simulink model "PI_continuo"  (R2012b)
settings: Solver=ode45  StartTime=0.0  StopTime=100  RelTol=1e-3
settings Model: Creator=Walter  LastModifiedBy=Walter

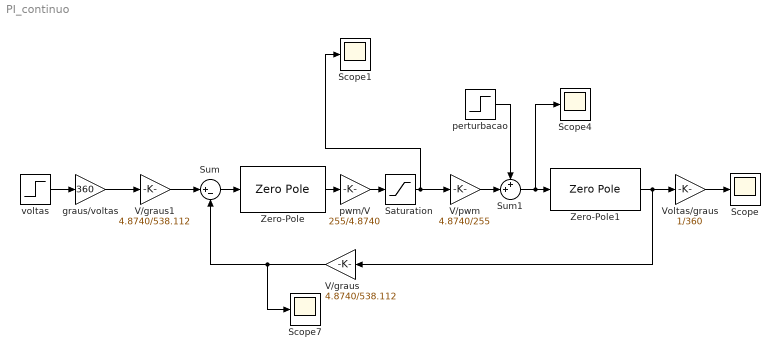
== system PI_continuo ==
  Saturation : Saturate  UpperLimit=255  LowerLimit=-255
  Scope{,1,4,7} (4 alike) : Scope
      Scope settings: TimeRange=60  YMin=2.5  YMax=6.5
      Scope1 settings: TimeRange=100
      Scope4 settings: SaveName=ScopeData4
      Scope7 settings: SaveName=ScopeData7
  Sum : Sum  Inputs=|+-
  Sum1 : Sum  Inputs=++|
  V/graus : Gain  Gain=4.8740/538.112
  V/graus1 : Gain  Gain=4.8740/538.112
  V/pwm : Gain  Gain=4.8740/255
  Voltas/graus : Gain  Gain=1/360
  Zero-Pole : ZeroPole  Zeros=[ -2.54]  Poles=[0]  Gain=[0.94]
  Zero-Pole1 : ZeroPole  Zeros=[]  Poles=[0 -35.7143]  Gain=[3943.0214]
  graus/voltas : Gain  Gain=360
  perturbacao : Step  After=0  SampleTime=0
  pwm/V : Gain  Gain=255/4.8740
  "voltas " : Step  Time=0  After=20  SampleTime=0
  wires:
  Sum/1 -> Zero-Pole/1
  pwm/V/1 -> Saturation/1
  Saturation/1 -> Scope1/1, V/pwm/1
  perturbacao/1 -> Sum1/1
  Sum1/1 -> Scope4/1, Zero-Pole1/1
  "voltas "/1 -> graus/voltas/1
  Zero-Pole1/1 -> Voltas/graus/1, V/graus/1
  V/graus/1 -> Scope7/1, Sum/2
  graus/voltas/1 -> V/graus1/1
  V/graus1/1 -> Sum/1
  V/pwm/1 -> Sum1/2
  Zero-Pole/1 -> pwm/V/1
  Voltas/graus/1 -> Scope/1
